simulink model "automata_learning"  (R2018a)
settings: Solver=FixedStepAuto  StartTime=0.0  StopTime=T  FixedStep=Ts  RelTol=1e-3
settings Model: Creator=xiaodong  LastModifiedBy=xiaodong

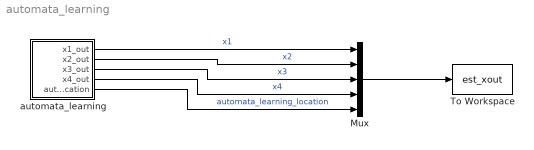
== system automata_learning ==
  Mux : Mux  Inputs=5
  To Workspace : ToWorkspace  VariableName=est_xout  SampleTime=-1
  automata_learning : Stateflow chart  TreatAsAtomicUnit=on
  wires:
  automata_learning/1(x1_out) -> Mux/1  "x1"
  automata_learning/2(x2_out) -> Mux/2  "x2"
  automata_learning/3(x3_out) -> Mux/3  "x3"
  automata_learning/4(x4_out) -> Mux/4  "x4"
  automata_learning/5(automata_learning_location) -> Mux/5  "automata_learning_location"
  Mux/1 -> To Workspace/1

== stateflow chart automata_learning/automata_learning ==
  settings: updateMethod=CONTINUOUS
  state loc1
    du:
    x1_dot = 0.0000000006366529256706548 * x2 - 0.00000000031713924399148346 * x1 + 1.0000001610969775 * x3 - 0.00000008079836904531165 * x4 - 0.00000013047198292679557;
    x2_dot = 0.0000000024185967664389074 * x2 - 0.000000001204724139644255 * x1 + 0.00000023563922261961995 * x3 + 0.9999998918119672 * x4 - 0.00000014620714961464942;
    x3_dot = 0.0036648094050590885 * x1 - 0.00735725130223841 * x2 - 1.2056134028025554 * x3 + 0.09965654588177131 * x4 + 1.204643648739875;
    x4_dot = 0.01069362314422051 * x1 - 0.021467875708481188 * x2 + 0.08362076555772546 * x3 - 1.2010023014154285 * x4 - 0.08645045392972861;
    x1_out=x1;
    x2_out=x2;
    x3_out=x3;
    x4_out=x4;
    automata_learning_location =1;
  state loc2
    du:
    x1_dot = 0.000000000000010316211919236548 * x2 - 0.00000000000008618674401024362 * x1 + 1.0000000742220436 * x3 - 0.0000000182751270854601 * x4 - 0.00000001827514557538974;
    x2_dot = 0.0000000000000008246170640003595 * x2 - 0.00000000000006457400296023534 * x1 - 0.000000018275142992657534 * x3 + 1.0000000742220436 * x4 + 0.00000007422372897921727;
    x3_dot = 0.00000000000000000009442668241800939 * x1 - 0.000000000000016248046627159078 * x2 - 1.200000090895628 * x3 + 0.10000002935248631 * x4 + 0.10000002935248631;
    x4_dot = 0.10000002935248631 * x3 - 0.0000000000000027641430754330486 * x2 - 0.0000000000000000000944266813068988 * x1 - 1.200000090895628 * x4 - 1.200000090895628;
    x1_out=x1;
    x2_out=x2;
    x3_out=x3;
    x4_out=x4;
    automata_learning_location =2;
  state loc3
    du:
    x1_dot = 0.00000000000002220446049250313 * x1 - 0.00000000000002437307871670544 * x2 + 1.0000000742220436 * x3 - 0.000000018275105504470066 * x4 - 0.00000006540655611174048;
    x2_dot = 1.0000000742220436 * x4 - 0.000000018275164446253812 * x3 - 0.00000000000001423696370617596 * x2 + 0.00000006540657883965378;
    x3_dot = 0.10000002935248631 * x4 - 1.200000090895628 * x3 - 0.00000000000002450188713740088 * x2 + 0.9192389005711448;
    x4_dot = 0.10000002935248631 * x3 - 0.000000000000007508935095362158 * x2 - 1.200000090895628 * x4 - 0.9192389005711448;
    x1_out=x1;
    x2_out=x2;
    x3_out=x3;
    x4_out=x4;
    automata_learning_location =3;
  state loc4
    du:
    x1_dot = 0.0;
    x2_dot = 0.0;
    x3_dot = 0.0;
    x4_dot = 0.0;
    x1_out=x1;
    x2_out=x2;
    x3_out=x3;
    x4_out=x4;
    automata_learning_location =4;
  state loc5
    du:
    x1_dot = 0.0000000006366529256706548 * x2 - 0.00000000031713924399148346 * x1 + 1.0000001610969775 * x3 - 0.00000008079836904531165 * x4 - 0.00000013047198292679557;
    x2_dot = 0.0000000024185967664389074 * x2 - 0.000000001204724139644255 * x1 + 0.00000023563922261961995 * x3 + 0.9999998918119672 * x4 - 0.00000014620714961464942;
    x3_dot = 0.0036648094050590885 * x1 - 0.00735725130223841 * x2 - 1.2056134028025554 * x3 + 0.09965654588177131 * x4 + 1.204643648739875;
    x4_dot = 0.01069362314422051 * x1 - 0.021467875708481188 * x2 + 0.08362076555772546 * x3 - 1.2010023014154285 * x4 - 0.08645045392972861;
    x1_out=x1;
    x2_out=x2;
    x3_out=x3;
    x4_out=x4;
    automata_learning_location =5;
  state loc6
    du:
    x1_dot = 0.000000000000010316211919236548 * x2 - 0.00000000000008618674401024362 * x1 + 1.0000000742220436 * x3 - 0.0000000182751270854601 * x4 - 0.00000001827514557538974;
    x2_dot = 0.0000000000000008246170640003595 * x2 - 0.00000000000006457400296023534 * x1 - 0.000000018275142992657534 * x3 + 1.0000000742220436 * x4 + 0.00000007422372897921727;
    x3_dot = 0.00000000000000000009442668241800939 * x1 - 0.000000000000016248046627159078 * x2 - 1.200000090895628 * x3 + 0.10000002935248631 * x4 + 0.10000002935248631;
    x4_dot = 0.10000002935248631 * x3 - 0.0000000000000027641430754330486 * x2 - 0.0000000000000000000944266813068988 * x1 - 1.200000090895628 * x4 - 1.200000090895628;
    x1_out=x1;
    x2_out=x2;
    x3_out=x3;
    x4_out=x4;
    automata_learning_location =6;
  state loc7
    du:
    x1_dot = 0.0;
    x2_dot = 0.0;
    x3_dot = 0.0;
    x4_dot = 0.0;
    x1_out=x1;
    x2_out=x2;
    x3_out=x3;
    x4_out=x4;
    automata_learning_location =7;
  loc3 -> loc6 [order 3] : [0.001934 * x2 - 0.4784 * x1 - 0.04486 * x3 + 0.01677 * x4 + 1.0 < 0.0]
  loc3 -> loc1 [order 1] : [0.008303 * x1 - 1.001 * x2 - 0.01661 * x3 + 0.01386 * x4 + 1.0 > 0.0]
  loc2 -> loc3 [order 1] : [0.002936 * x2 - 1.006 * x1 + 0.01943 * x3 - 0.00276 * x4 + 1.0 < 0.0]
  loc6 -> loc7 : [0.005433 * x1 - 0.971 * x2 - 0.01764 * x3 + 0.05212 * x4 + 1.0 > 0.0]
  loc1 -> loc2 [order 1] : [0.004217 * x1 - 0.9989 * x2 - 0.01078 * x3 + 0.021 * x4 + 1.0 < 0.0]
  (default) -> loc1 : {x1 = x_init(1);
      | x2 = x_init(2);
      | x3 = x_init(3);
      | x4 = x_init(4);}
  loc2 -> loc1 [order 2] : [0.001144 * x1 - 1.007 * x2 + 0.01591 * x3 + 0.0126 * x4 + 1.0 > 0.0]
  loc1 -> loc4 [order 2] : [0.006683 * x3 - 0.0009015 * x2 - 0.5018 * x1 - 0.002991 * x4 + 1.0 < 0.0]
  loc3 -> loc5 [order 2] : [0.003064 * x3 - 0.4986 * x2 - 0.005362 * x1 + 0.01004 * x4 + 1.0 < 0.0]
  loc5 -> loc6 : [0.002993 * x4 - 0.004894 * x2 - 0.0009216 * x3 - 0.4904 * x1 + 1.0 < 0.0]
  data: x1_out output; x1 local; x2_out output; x2 local; x3_out output; x3 local; x4_out output; x4 local; automata_learning_location output; x_init constant double size=4 =x_init
  data x1 settings: updateMethod=SF_CONTINUOUS_TIME_DATA
  data x2 settings: updateMethod=SF_CONTINUOUS_TIME_DATA
  data x3 settings: updateMethod=SF_CONTINUOUS_TIME_DATA
  data x4 settings: updateMethod=SF_CONTINUOUS_TIME_DATA
